simulink model "Md61Md62CalibSet"  (R2018b)
settings: Solver=FixedStepDiscrete  StartTime=0.0  StopTime=10.0  FixedStep=0.01  RelTol=1e-3
undefined symbols (not defined in the file or in its folder): KeSMSuFirstRwStBackPosDelta_Val, KeSMSuFirstRwStCushFoldPosDelta_Val, KeSMSuFirstRwStFwdBkwdPosDelta_Val, KeSMSuThrdRwCushFoldPosDelta_Val, KeSMSwAcsMd30PassStBkReclnUpwdDnwdPos1_Val, KeSMSwAcsMd30PassStBkReclnUpwdDnwdPos1Max_Val, KeSMSwAcsMd30PassStBkReclnUpwdDnwdPos1Min_Val, KeSMSwAcsMd30PassStFldUpwdDnwdPos1_Val, KeSMSwAcsMd30PassStFrwdBkwdPos1_Val, KeSMSwAcsMd30PassStFrwdBkwdPos1Max_Val, KeSMSwAcsMd30PassStFrwdBkwdPos1Min_Val, KeSMSwSeatBkLimitPos_Val, KeSMSwSeatBkLimitPosDelt_Val
libraries: StIsPosChkLib x2
(part 2 of 5)

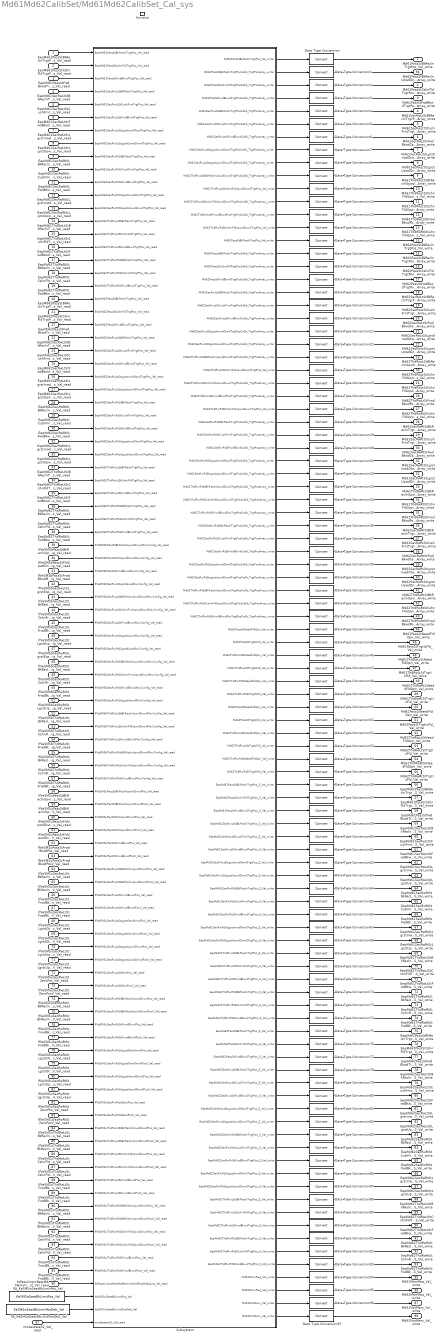
== system Md61Md62CalibSet/Md61Md62CalibSet_Cal_sys ==
  EepMd61PassStBkReclnTrgtPos_Val_read : Inport
  EepMd61PassStCshnFldTrgtPos_Val_read : Inport  Port=2
  EepMd61PassStFwdBkwdTrgtPos_Val_read : Inport  Port=3
  EepMd61SecRwLtStBkReclnTrgtPos_Val_read : Inport  Port=4
  EepMd61SecRwLtStCushFrntTrgtPos_Val_read : Inport  Port=5
  EepMd61SecRwLtStFwdBkwdTrgtPos_Val_read : Inport  Port=6
  EepMd61SecRwLtStLgrstInwdOtwdTrgtPos_Val_read : Inport  Port=7
  EepMd61SecRwLtStLgrstUpwdDnwdTrgtPos_Val_read : Inport  Port=8
  EepMd61SecRwRtStBkReclnTrgtPos_Val_read : Inport  Port=9
  EepMd61SecRwRtStCushFrntTrgtPos_Val_read : Inport  Port=10
  EepMd61SecRwRtStFwdBkwdTrgtPos_Val_read : Inport  Port=11
  EepMd61SecRwRtStLgrstInwdOtwdTrgtPos_Val_read : Inport  Port=12
  EepMd61SecRwRtStLgrstUpwdDnwdTrgtPos_Val_read : Inport  Port=13
  EepMd61ThdRwLtStBkReclnTrgtPos_Val_read : Inport  Port=14
  EepMd61ThdRwLtStCshnFldTrgtPos_Val_read : Inport  Port=15
  EepMd61ThdRwLtStFwdBkwdTrgtPos_Val_read : Inport  Port=16
  EepMd61ThdRwRtStBkReclnTrgtPos_Val_read : Inport  Port=17
  EepMd61ThdRwRtStCshnFldTrgtPos_Val_read : Inport  Port=18
  EepMd61ThdRwRtStFwdBkwdTrgtPos_Val_read : Inport  Port=19
  EepMd62PassStBkReclnTrgtPos_Val_read : Inport  Port=20
  EepMd62PassStCshnFldTrgtPos_Val_read : Inport  Port=21
  EepMd62PassStFwdBkwdTrgtPos_Val_read : Inport  Port=22
  EepMd62SecRwLtStBkReclnTrgtPos_Val_read : Inport  Port=23
  EepMd62SecRwLtStCushFrntTrgtPos_Val_read : Inport  Port=24
  EepMd62SecRwLtStFwdBkwdTrgtPos_Val_read : Inport  Port=25
  EepMd62SecRwLtStLgrstInwdOtwdTrgtPos_Val_read : Inport  Port=26
  EepMd62SecRwLtStLgrstUpwdDnwdTrgtPos_Val_read : Inport  Port=27
  EepMd62SecRwRtStBkReclnTrgtPos_Val_read : Inport  Port=28
  EepMd62SecRwRtStCushFrntTrgtPos_Val_read : Inport  Port=29
  EepMd62SecRwRtStFwdBkwdTrgtPos_Val_read : Inport  Port=30
  EepMd62SecRwRtStLgrstInwdOtwdTrgtPos_Val_read : Inport  Port=31
  EepMd62SecRwRtStLgrstUpwdDnwdTrgtPos_Val_read : Inport  Port=32
  EepMd62ThdRwLtStBkReclnTrgtPos_Val_read : Inport  Port=33
  EepMd62ThdRwLtStCshnFldTrgtPos_Val_read : Inport  Port=34
  EepMd62ThdRwLtStFwdBkwdTrgtPos_Val_read : Inport  Port=35
  EepMd62ThdRwRtStBkReclnTrgtPos_Val_read : Inport  Port=36
  EepMd62ThdRwRtStCshnFldTrgtPos_Val_read : Inport  Port=37
  EepMd62ThdRwRtStFwdBkwdTrgtPos_Val_read : Inport  Port=38
  IfVeSMSbPassStBkReclnUpwdDnwdMovConfig_Val_read : Inport  Port=39
  IfVeSMSbPassStFldUpwdDnwdMovConfig_Val_read : Inport  Port=40
  IfVeSMSbPassStFrwdBkwdMovConfig_Val_read : Inport  Port=41
  IfVeSMSbSecRwLtSLgrstExpdMovConfig_Val_read : Inport  Port=42
  IfVeSMSbSecRwLtStBkReclnUpwdDnwdMovConfig_Val_read : Inport  Port=43
  IfVeSMSbSecRwLtStCshnFrntUpwdDnwdMovConfig_Val_read : Inport  Port=44
  IfVeSMSbSecRwLtStFrwdBkwdMovConfig_Val_read : Inport  Port=45
  IfVeSMSbSecRwLtStLgrstUpwdMovConfig_Val_read : Inport  Port=46
  IfVeSMSbSecRwRtSLgrstExpdMovConfig_Val_read : Inport  Port=47
  IfVeSMSbSecRwRtStBkReclnUpwdDnwdMovConfig_Val_read : Inport  Port=48
  IfVeSMSbSecRwRtStCshnFrntUpwdDnwdMovConfig_Val_read : Inport  Port=49
  IfVeSMSbSecRwRtStFrwdBkwdMovConfig_Val_read : Inport  Port=50
  IfVeSMSbSecRwRtStLgrstUpwdMovConfig_Val_read : Inport  Port=51
  IfVeSMSbThdRwLtStBkReclnUpwdDnwdMovConfig_Val_read : Inport  Port=52
  IfVeSMSbThdRwLtStCshnFldUpwdDnwdMovConfig_Val_read : Inport  Port=53
  IfVeSMSbThdRwLtStFrwdBkwdMovConfig_Val_read : Inport  Port=54
  IfVeSMSbThdRwRtStBkReclnUpwdDnwdMovConfig_Val_read : Inport  Port=55
  IfVeSMSbThdRwRtStCshnFldUpwdDnwdMovConfig_Val_read : Inport  Port=56
  IfVeSMSbThdRwRtStFrwdBkwdMovConfig_Val_read : Inport  Port=57
  IfVeSMSuPassStBkReclnUpwdDnwdPos_Val_read : Inport  Port=58
  IfVeSMSuPassStBkReclnUpwdDnwdPosV_Val_read : Inport  Port=59
  IfVeSMSuPassStFldUpwdDnwdPos_Val_read : Inport  Port=60
  IfVeSMSuPassStFldUpwdDnwdPosV_Val_read : Inport  Port=61
  IfVeSMSuPassStFrwdBkwdPos_Val_read : Inport  Port=62
  IfVeSMSuPassStFrwdBkwdPosV_Val_read : Inport  Port=63
  IfVeSMSuSecRwLtStBkReclnUpwdDnwdPos_Val_read : Inport  Port=64
  IfVeSMSuSecRwLtStBkReclnUpwdDnwdPosV_Val_read : Inport  Port=65
  IfVeSMSuSecRwLtStFrwdBkwdPos_Val_read : Inport  Port=66
  IfVeSMSuSecRwLtStFrwdBkwdPosV_Val_read : Inport  Port=67
  IfVeSMSuSecRwLtStLgrstOtwdInwdPos_Val_read : Inport  Port=68
  IfVeSMSuSecRwLtStLgrstOtwdInwdPosV_Val_read : Inport  Port=69
  IfVeSMSuSecRwLtStLgrstUpwdDnwdPos_Val_read : Inport  Port=70
  IfVeSMSuSecRwLtStLgrstUpwdDnwdPosV_Val_read : Inport  Port=71
  IfVeSMSuSecRwLtStZeroPos_Val_read : Inport  Port=72
  IfVeSMSuSecRwLtStZeroPosV_Val_read : Inport  Port=73
  IfVeSMSuSecRwRtStBkReclnUpwdDnwdPos_Val_read : Inport  Port=74
  IfVeSMSuSecRwRtStBkReclnUpwdDnwdPosV_Val_read : Inport  Port=75
  IfVeSMSuSecRwRtStFrwdBkwdPos_Val_read : Inport  Port=76
  IfVeSMSuSecRwRtStFrwdBkwdPosV_Val_read : Inport  Port=77
  IfVeSMSuSecRwRtStLgrstOtwdInwdPos_Val_read : Inport  Port=78
  IfVeSMSuSecRwRtStLgrstOtwdInwdPosV_Val_read : Inport  Port=79
  IfVeSMSuSecRwRtStLgrstUpwdDnwdPos_Val_read : Inport  Port=80
  IfVeSMSuSecRwRtStLgrstUpwdDnwdPosV_Val_read : Inport  Port=81
  IfVeSMSuSecRwRtStZeroPos_Val_read : Inport  Port=82
  IfVeSMSuSecRwRtStZeroPosV_Val_read : Inport  Port=83
  IfVeSMSuThdRwLtStBkReclnUpwdDnwdPos_Val_read : Inport  Port=84
  IfVeSMSuThdRwLtStBkReclnUpwdDnwdPosV_Val_read : Inport  Port=85
  IfVeSMSuThdRwLtStCshnFldUpwdDnwdPos_Val_read : Inport  Port=86
  IfVeSMSuThdRwLtStCshnFldUpwdDnwdPosV_Val_read : Inport  Port=87
  IfVeSMSuThdRwLtStFrwdBkwdPos_Val_read : Inport  Port=88
  IfVeSMSuThdRwLtStFrwdBkwdPosV_Val_read : Inport  Port=89
  IfVeSMSuThdRwRtStBkReclnUpwdDnwdPos_Val_read : Inport  Port=90
  IfVeSMSuThdRwRtStBkReclnUpwdDnwdPosV_Val_read : Inport  Port=91
  IfVeSMSuThdRwRtStCshnFldUpwdDnwdPos_Val_read : Inport  Port=92
  IfVeSMSuThdRwRtStCshnFldUpwdDnwdPosV_Val_read : Inport  Port=93
  IfVeSMSuThdRwRtStFrwdBkwdPos_Val_read : Inport  Port=94
  IfVeSMSuThdRwRtStFrwdBkwdPosV_Val_read : Inport  Port=95
  StPassCmprtRestMdMemVirtCtrlReqMdadjust_Val_read : Inport  Port=96
  modestate32_Val_read : Inport  Port=97
  function : TriggerPort  TriggerType=function-call  IsSimulinkFunction=on  FunctionName=Md61Md62CalibSet_Cal  VariantControl=(inherit)
  Data Type Conversion{,1..97} (98 alike) : DataTypeConversion
  PA_KeSMSwSeatBkLimitPosDelt_Val : Constant  Value=KeSMSwSeatBkLimitPosDelt_Val
  PA_KeSMSwSeatBkLimitPos_Val : Constant  Value=KeSMSwSeatBkLimitPos_Val
  Subsystem : Subsystem
  Md61PassStBkReclnTrgtPos_Val_write : Outport
      settings: EnsureOutportIsVirtual=on
  Md61PassStCshnFldTrgtPosCalib_TrgtPosArray_write : Outport  Port=2
      settings: EnsureOutportIsVirtual=on
  Md61PassStFwdBkwdTrgtPosCalib_TrgtPosArray_write : Outport  Port=3
      settings: EnsureOutportIsVirtual=on
  Md61SecRwLtStBkReclnTrgtPosCalib_TrgtPosArray_write : Outport  Port=4
      settings: EnsureOutportIsVirtual=on
  Md61SecRwLtStCushFrntTrgtPosCalib_TrgtPosArray_write : Outport  Port=5
      settings: EnsureOutportIsVirtual=on
  Md61SecRwLtStFwdBkwdCalib_TrgtPosArray_write : Outport  Port=6
      settings: EnsureOutportIsVirtual=on
  Md61SecRwLtStLgrstInwdOtwdTrgtPosCalib_TrgtPosArray_write : Outport  Port=7
      settings: EnsureOutportIsVirtual=on
  Md61SecRwLtStLgrstUpwdDnwdTrgtPosCalib_TrgtPosArray_write : Outport  Port=8
      settings: EnsureOutportIsVirtual=on
  Md61ThdRwLtStBkReclnUpwdDnwdTrgtPosCalib_TrgtPosArray_write : Outport  Port=9
      settings: EnsureOutportIsVirtual=on
  Md61ThdRwLtStCshnFldUpwdDnwdTrgtPos_Val_write : Outport  Port=10
      settings: EnsureOutportIsVirtual=on
  Md61ThdRwLtStCshnFldUpwdDnwdTrgtPosCalib_TrgtPosArray_write : Outport  Port=11
      settings: EnsureOutportIsVirtual=on
  Md61ThdRwLtStFrwdBkwdPosTrgtPosCalib_TrgtPosArray_write : Outport  Port=12
      settings: EnsureOutportIsVirtual=on
  Md61ThdRwRtStCshnFldUpwdDnwdTrgtPos_Val_write : Outport  Port=13
      settings: EnsureOutportIsVirtual=on
  Md62PassStBkReclnTrgtPos_Val_write : Outport  Port=14
      settings: EnsureOutportIsVirtual=on
  Md62PassStBkReclnTrgtPosCalib_TrgtPosArray_write : Outport  Port=15
      settings: EnsureOutportIsVirtual=on
  Md62PassStCshnFldTrgtPosCalib_TrgtPosArray_write : Outport  Port=16
      settings: EnsureOutportIsVirtual=on
  Md62PassStFwdBkwdTrgtPosCalib_TrgtPosArray_write : Outport  Port=17
      settings: EnsureOutportIsVirtual=on
  Md62SecRwLtStBkReclnTrgtPosCalib_TrgtPosArray_write : Outport  Port=18
      settings: EnsureOutportIsVirtual=on
  Md62SecRwLtStCushFrntTrgtPosCalib_TrgtPosArray_write : Outport  Port=19
      settings: EnsureOutportIsVirtual=on
  Md62SecRwLtStFwdBkwdCalib_TrgtPosArray_write : Outport  Port=20
      settings: EnsureOutportIsVirtual=on
  Md62SecRwLtStLgrstInwdOtwdTrgtPosCalib_TrgtPosArray_write : Outport  Port=21
      settings: EnsureOutportIsVirtual=on
  Md62SecRwLtStLgrstUpwdDnwdTrgtPosCalib_TrgtPosArray_write : Outport  Port=22
      settings: EnsureOutportIsVirtual=on
  Md62ThdRwLtStBkReclnUpwdDnwdTrgtPosCalib_TrgtPosArray_write : Outport  Port=23
      settings: EnsureOutportIsVirtual=on
  Md62ThdRwLtStCshnFldUpwdDnwdTrgtPos_Val_write : Outport  Port=24
      settings: EnsureOutportIsVirtual=on
  Md62ThdRwLtStCshnFldUpwdDnwdTrgtPosCalib_TrgtPosArray_write : Outport  Port=25
      settings: EnsureOutportIsVirtual=on
  Md62ThdRwLtStFrwdBkwdPosTrgtPosCalib_TrgtPosArray_write : Outport  Port=26
      settings: EnsureOutportIsVirtual=on
  Md62ThdRwRtStCshnFldUpwdDnwdTrgtPos_Val_write : Outport  Port=27
      settings: EnsureOutportIsVirtual=on
  Md61SecRwRtStBkReclnTrgtPosCalib_TrgtPosArray_write : Outport  Port=28
      settings: EnsureOutportIsVirtual=on
  Md61SecRwRtStCushFrntTrgtPosCalib_TrgtPosArray_write : Outport  Port=29
      settings: EnsureOutportIsVirtual=on
  Md61SecRwRtStFwdBkwdCalib_TrgtPosArray_write : Outport  Port=30
      settings: EnsureOutportIsVirtual=on
  Md61SecRwRtStLgrstInwdOtwdTrgtPosCalib_TrgtPosArray_write : Outport  Port=31
      settings: EnsureOutportIsVirtual=on
  Md61SecRwRtStLgrstUpwdDnwdTrgtPosCalib_TrgtPosArray_write : Outport  Port=32
      settings: EnsureOutportIsVirtual=on
  Md61ThdRwRtStBkReclnUpwdDnwdTrgtPosCalib_TrgtPosArray_write : Outport  Port=33
      settings: EnsureOutportIsVirtual=on
  Md61ThdRwRtStCshnFldUpwdDnwdTrgtPosCalib_TrgtPosArray_write : Outport  Port=34
      settings: EnsureOutportIsVirtual=on
  Md61ThdRwRtStFrwdBkwdPosTrgtPosCalib_TrgtPosArray_write : Outport  Port=35
      settings: EnsureOutportIsVirtual=on
  Md62SecRwRtStBkReclnTrgtPosCalib_TrgtPosArray_write : Outport  Port=36
      settings: EnsureOutportIsVirtual=on
  Md62SecRwRtStCushFrntTrgtPosCalib_TrgtPosArray_write : Outport  Port=37
      settings: EnsureOutportIsVirtual=on
  Md62SecRwRtStFwdBkwdCalib_TrgtPosArray_write : Outport  Port=38
      settings: EnsureOutportIsVirtual=on
  Md62SecRwRtStLgrstInwdOtwdTrgtPosCalib_TrgtPosArray_write : Outport  Port=39
      settings: EnsureOutportIsVirtual=on
  Md62SecRwRtStLgrstUpwdDnwdTrgtPosCalib_TrgtPosArray_write : Outport  Port=40
      settings: EnsureOutportIsVirtual=on
  Md62ThdRwRtStBkReclnUpwdDnwdTrgtPosCalib_TrgtPosArray_write : Outport  Port=41
      settings: EnsureOutportIsVirtual=on
  Md62ThdRwRtStCshnFldUpwdDnwdTrgtPosCalib_TrgtPosArray_write : Outport  Port=42
      settings: EnsureOutportIsVirtual=on
  Md62ThdRwRtStFrwdBkwdPosTrgtPosCalib_TrgtPosArray_write : Outport  Port=43
      settings: EnsureOutportIsVirtual=on
  Md61PassStNeedFldOpn_Val_write : Outport  Port=44
      settings: EnsureOutportIsVirtual=on
  Md61PassStTrgtIsFld_Val_write : Outport  Port=45
      settings: EnsureOutportIsVirtual=on
  Md61ThdRwLtStNeedFldOpn_Val_write : Outport  Port=46
      settings: EnsureOutportIsVirtual=on
  Md61ThdRwLtStTrgtIsFld_Val_write : Outport  Port=47
      settings: EnsureOutportIsVirtual=on
  Md61ThdRwRtStNeedFldOpn_Val_write : Outport  Port=48
      settings: EnsureOutportIsVirtual=on
  Md61ThdRwRtStTrgtIsFld_Val_write : Outport  Port=49
      settings: EnsureOutportIsVirtual=on
  Md62PassStNeedFldOpn_Val_write : Outport  Port=50
      settings: EnsureOutportIsVirtual=on
  Md62PassStTrgtIsFld_Val_write : Outport  Port=51
      settings: EnsureOutportIsVirtual=on
  Md62ThdRwLtStNeedFldOpn_Val_write : Outport  Port=52
      settings: EnsureOutportIsVirtual=on
  Md62ThdRwLtStTrgtIsFld_Val_write : Outport  Port=53
      settings: EnsureOutportIsVirtual=on
  Md62ThdRwRtStNeedFldOpn_Val_write : Outport  Port=54
      settings: EnsureOutportIsVirtual=on
  Md62ThdRwRtStTrgtIsFld_Val_write : Outport  Port=55
      settings: EnsureOutportIsVirtual=on
  EepMd61PassStBkReclnTrgtPos_S_Val_write : Outport  Port=56
      settings: EnsureOutportIsVirtual=on
  EepMd61PassStCshnFldTrgtPos_S_Val_write : Outport  Port=57
      settings: EnsureOutportIsVirtual=on
  EepMd61PassStFwdBkwdTrgtPos_S_Val_write : Outport  Port=58
      settings: EnsureOutportIsVirtual=on
  EepMd61SecRwLtStBkReclnTrgtPos_S_Val_write : Outport  Port=59
      settings: EnsureOutportIsVirtual=on
  EepMd61SecRwLtStCushFrntTrgtPos_S_Val_write : Outport  Port=60
      settings: EnsureOutportIsVirtual=on
  EepMd61SecRwLtStFwdBkwdTrgtPos_S_Val_write : Outport  Port=61
      settings: EnsureOutportIsVirtual=on
  EepMd61SecRwLtStLgrstInwdOtwdTrgtPos_S_Val_write : Outport  Port=62
      settings: EnsureOutportIsVirtual=on
  EepMd61SecRwLtStLgrstUpwdDnwdTrgtPos_S_Val_write : Outport  Port=63
      settings: EnsureOutportIsVirtual=on
  EepMd61SecRwRtStBkReclnTrgtPos_S_Val_write : Outport  Port=64
      settings: EnsureOutportIsVirtual=on
  EepMd61SecRwRtStCushFrntTrgtPos_S_Val_write : Outport  Port=65
      settings: EnsureOutportIsVirtual=on
  EepMd61SecRwRtStFwdBkwdTrgtPos_S_Val_write : Outport  Port=66
      settings: EnsureOutportIsVirtual=on
  EepMd61SecRwRtStLgrstInwdOtwdTrgtPos_S_Val_write : Outport  Port=67
      settings: EnsureOutportIsVirtual=on
  EepMd61SecRwRtStLgrstUpwdDnwdTrgtPos_S_Val_write : Outport  Port=68
      settings: EnsureOutportIsVirtual=on
  EepMd61ThdRwLtStBkReclnTrgtPos_S_Val_write : Outport  Port=69
      settings: EnsureOutportIsVirtual=on
  EepMd61ThdRwLtStCshnFldTrgtPos_S_Val_write : Outport  Port=70
      settings: EnsureOutportIsVirtual=on
  EepMd61ThdRwLtStFwdBkwdTrgtPos_S_Val_write : Outport  Port=71
      settings: EnsureOutportIsVirtual=on
  EepMd61ThdRwRtStBkReclnTrgtPos_S_Val_write : Outport  Port=72
      settings: EnsureOutportIsVirtual=on
  EepMd61ThdRwRtStCshnFldTrgtPos_S_Val_write : Outport  Port=73
      settings: EnsureOutportIsVirtual=on
  EepMd61ThdRwRtStFwdBkwdTrgtPos_S_Val_write : Outport  Port=74
      settings: EnsureOutportIsVirtual=on
  EepMd62PassStBkReclnTrgtPos_S_Val_write : Outport  Port=75
      settings: EnsureOutportIsVirtual=on
  EepMd62PassStCshnFldTrgtPos_S_Val_write : Outport  Port=76
      settings: EnsureOutportIsVirtual=on
  EepMd62PassStFwdBkwdTrgtPos_S_Val_write : Outport  Port=77
      settings: EnsureOutportIsVirtual=on
  EepMd62SecRwLtStBkReclnTrgtPos_S_Val_write : Outport  Port=78
      settings: EnsureOutportIsVirtual=on
  EepMd62SecRwLtStCushFrntTrgtPos_S_Val_write : Outport  Port=79
      settings: EnsureOutportIsVirtual=on
  EepMd62SecRwLtStFwdBkwdTrgtPos_S_Val_write : Outport  Port=80
      settings: EnsureOutportIsVirtual=on
  EepMd62SecRwLtStLgrstInwdOtwdTrgtPos_S_Val_write : Outport  Port=81
      settings: EnsureOutportIsVirtual=on
  EepMd62SecRwLtStLgrstUpwdDnwdTrgtPos_S_Val_write : Outport  Port=82
      settings: EnsureOutportIsVirtual=on
  EepMd62SecRwRtStBkReclnTrgtPos_S_Val_write : Outport  Port=83
      settings: EnsureOutportIsVirtual=on
  EepMd62SecRwRtStCushFrntTrgtPos_S_Val_write : Outport  Port=84
      settings: EnsureOutportIsVirtual=on
  EepMd62SecRwRtStFwdBkwdTrgtPos_S_Val_write : Outport  Port=85
      settings: EnsureOutportIsVirtual=on
  EepMd62SecRwRtStLgrstInwdOtwdTrgtPos_S_Val_write : Outport  Port=86
      settings: EnsureOutportIsVirtual=on
  EepMd62SecRwRtStLgrstUpwdDnwdTrgtPos_S_Val_write : Outport  Port=87
      settings: EnsureOutportIsVirtual=on
  EepMd62ThdRwLtStBkReclnTrgtPos_S_Val_write : Outport  Port=88
      settings: EnsureOutportIsVirtual=on
  EepMd62ThdRwLtStCshnFldTrgtPos_S_Val_write : Outport  Port=89
      settings: EnsureOutportIsVirtual=on
  EepMd62ThdRwLtStFwdBkwdTrgtPos_S_Val_write : Outport  Port=90
      settings: EnsureOutportIsVirtual=on
  EepMd62ThdRwRtStBkReclnTrgtPos_S_Val_write : Outport  Port=91
      settings: EnsureOutportIsVirtual=on
  EepMd62ThdRwRtStCshnFldTrgtPos_S_Val_write : Outport  Port=92
      settings: EnsureOutportIsVirtual=on
  EepMd62ThdRwRtStFwdBkwdTrgtPos_S_Val_write : Outport  Port=93
      settings: EnsureOutportIsVirtual=on
  Md61PassStBkReclnUpwdDnwdTrgtPosCalib_TrgtPosArray_write : Outport  Port=94
      settings: EnsureOutportIsVirtual=on
  Md61MemReq_Val_write : Outport  Port=95
      settings: EnsureOutportIsVirtual=on
  Md62MemReq_Val_write : Outport  Port=96
      settings: EnsureOutportIsVirtual=on
  Md61NotMem_Val_write : Outport  Port=97
      settings: EnsureOutportIsVirtual=on
  Md62NotMem_Val_write : Outport  Port=98
      settings: EnsureOutportIsVirtual=on
  wires:
  EepMd61PassStBkReclnTrgtPos_Val_read/1 -> Subsystem/1(EepMd61PassStBkReclnTrgtPos_Val_read)
  EepMd61PassStCshnFldTrgtPos_Val_read/1 -> Subsystem/2(EepMd61PassStCshnFldTrgtPos_Val_read)
  EepMd61PassStFwdBkwdTrgtPos_Val_read/1 -> Subsystem/3(EepMd61PassStFwdBkwdTrgtPos_Val_read)
  EepMd61SecRwLtStBkReclnTrgtPos_Val_read/1 -> Subsystem/4(EepMd61SecRwLtStBkReclnTrgtPos_Val_read)
  EepMd61SecRwLtStCushFrntTrgtPos_Val_read/1 -> Subsystem/5(EepMd61SecRwLtStCushFrntTrgtPos_Val_read)
  EepMd61SecRwLtStFwdBkwdTrgtPos_Val_read/1 -> Subsystem/6(EepMd61SecRwLtStFwdBkwdTrgtPos_Val_read)
  EepMd61SecRwLtStLgrstInwdOtwdTrgtPos_Val_read/1 -> Subsystem/7(EepMd61SecRwLtStLgrstInwdOtwdTrgtPos_Val_read)
  EepMd61SecRwLtStLgrstUpwdDnwdTrgtPos_Val_read/1 -> Subsystem/8(EepMd61SecRwLtStLgrstUpwdDnwdTrgtPos_Val_read)
  EepMd61SecRwRtStBkReclnTrgtPos_Val_read/1 -> Subsystem/9(EepMd61SecRwRtStBkReclnTrgtPos_Val_read)
  EepMd61SecRwRtStCushFrntTrgtPos_Val_read/1 -> Subsystem/10(EepMd61SecRwRtStCushFrntTrgtPos_Val_read)
  EepMd61SecRwRtStFwdBkwdTrgtPos_Val_read/1 -> Subsystem/11(EepMd61SecRwRtStFwdBkwdTrgtPos_Val_read)
  EepMd61SecRwRtStLgrstInwdOtwdTrgtPos_Val_read/1 -> Subsystem/12(EepMd61SecRwRtStLgrstInwdOtwdTrgtPos_Val_read)
  EepMd61SecRwRtStLgrstUpwdDnwdTrgtPos_Val_read/1 -> Subsystem/13(EepMd61SecRwRtStLgrstUpwdDnwdTrgtPos_Val_read)
  EepMd61ThdRwLtStBkReclnTrgtPos_Val_read/1 -> Subsystem/14(EepMd61ThdRwLtStBkReclnTrgtPos_Val_read)
  EepMd61ThdRwLtStCshnFldTrgtPos_Val_read/1 -> Subsystem/15(EepMd61ThdRwLtStCshnFldTrgtPos_Val_read)
  EepMd61ThdRwLtStFwdBkwdTrgtPos_Val_read/1 -> Subsystem/16(EepMd61ThdRwLtStFwdBkwdTrgtPos_Val_read)
  EepMd61ThdRwRtStBkReclnTrgtPos_Val_read/1 -> Subsystem/17(EepMd61ThdRwRtStBkReclnTrgtPos_Val_read)
  EepMd61ThdRwRtStCshnFldTrgtPos_Val_read/1 -> Subsystem/18(EepMd61ThdRwRtStCshnFldTrgtPos_Val_read)
  EepMd61ThdRwRtStFwdBkwdTrgtPos_Val_read/1 -> Subsystem/19(EepMd61ThdRwRtStFwdBkwdTrgtPos_Val_read)
  EepMd62PassStBkReclnTrgtPos_Val_read/1 -> Subsystem/20(EepMd62PassStBkReclnTrgtPos_Val_read)
  EepMd62PassStCshnFldTrgtPos_Val_read/1 -> Subsystem/21(EepMd62PassStCshnFldTrgtPos_Val_read)
  EepMd62PassStFwdBkwdTrgtPos_Val_read/1 -> Subsystem/22(EepMd62PassStFwdBkwdTrgtPos_Val_read)
  EepMd62SecRwLtStBkReclnTrgtPos_Val_read/1 -> Subsystem/23(EepMd62SecRwLtStBkReclnTrgtPos_Val_read)
  EepMd62SecRwLtStCushFrntTrgtPos_Val_read/1 -> Subsystem/24(EepMd62SecRwLtStCushFrntTrgtPos_Val_read)
  EepMd62SecRwLtStFwdBkwdTrgtPos_Val_read/1 -> Subsystem/25(EepMd62SecRwLtStFwdBkwdTrgtPos_Val_read)
  EepMd62SecRwLtStLgrstInwdOtwdTrgtPos_Val_read/1 -> Subsystem/26(EepMd62SecRwLtStLgrstInwdOtwdTrgtPos_Val_read)
  EepMd62SecRwLtStLgrstUpwdDnwdTrgtPos_Val_read/1 -> Subsystem/27(EepMd62SecRwLtStLgrstUpwdDnwdTrgtPos_Val_read)
  EepMd62SecRwRtStBkReclnTrgtPos_Val_read/1 -> Subsystem/28(EepMd62SecRwRtStBkReclnTrgtPos_Val_read)
  EepMd62SecRwRtStCushFrntTrgtPos_Val_read/1 -> Subsystem/29(EepMd62SecRwRtStCushFrntTrgtPos_Val_read)
  EepMd62SecRwRtStFwdBkwdTrgtPos_Val_read/1 -> Subsystem/30(EepMd62SecRwRtStFwdBkwdTrgtPos_Val_read)
  EepMd62SecRwRtStLgrstInwdOtwdTrgtPos_Val_read/1 -> Subsystem/31(EepMd62SecRwRtStLgrstInwdOtwdTrgtPos_Val_read)
  EepMd62SecRwRtStLgrstUpwdDnwdTrgtPos_Val_read/1 -> Subsystem/32(EepMd62SecRwRtStLgrstUpwdDnwdTrgtPos_Val_read)
  EepMd62ThdRwLtStBkReclnTrgtPos_Val_read/1 -> Subsystem/33(EepMd62ThdRwLtStBkReclnTrgtPos_Val_read)
  EepMd62ThdRwLtStCshnFldTrgtPos_Val_read/1 -> Subsystem/34(EepMd62ThdRwLtStCshnFldTrgtPos_Val_read)
  EepMd62ThdRwLtStFwdBkwdTrgtPos_Val_read/1 -> Subsystem/35(EepMd62ThdRwLtStFwdBkwdTrgtPos_Val_read)
  EepMd62ThdRwRtStBkReclnTrgtPos_Val_read/1 -> Subsystem/36(EepMd62ThdRwRtStBkReclnTrgtPos_Val_read)
  EepMd62ThdRwRtStCshnFldTrgtPos_Val_read/1 -> Subsystem/37(EepMd62ThdRwRtStCshnFldTrgtPos_Val_read)
  EepMd62ThdRwRtStFwdBkwdTrgtPos_Val_read/1 -> Subsystem/38(EepMd62ThdRwRtStFwdBkwdTrgtPos_Val_read)
  IfVeSMSbPassStBkReclnUpwdDnwdMovConfig_Val_read/1 -> Subsystem/39(IfVeSMSbPassStBkReclnUpwdDnwdMovConfig_Val_read)
  IfVeSMSbPassStFldUpwdDnwdMovConfig_Val_read/1 -> Subsystem/40(IfVeSMSbPassStFldUpwdDnwdMovConfig_Val_read)
  IfVeSMSbPassStFrwdBkwdMovConfig_Val_read/1 -> Subsystem/41(IfVeSMSbPassStFrwdBkwdMovConfig_Val_read)
  IfVeSMSbSecRwLtSLgrstExpdMovConfig_Val_read/1 -> Subsystem/42(IfVeSMSbSecRwLtSLgrstExpdMovConfig_Val_read)
  IfVeSMSbSecRwLtStBkReclnUpwdDnwdMovConfig_Val_read/1 -> Subsystem/43(IfVeSMSbSecRwLtStBkReclnUpwdDnwdMovConfig_Val_read)
  IfVeSMSbSecRwLtStCshnFrntUpwdDnwdMovConfig_Val_read/1 -> Subsystem/44(IfVeSMSbSecRwLtStCshnFrntUpwdDnwdMovConfig_Val_read)
  IfVeSMSbSecRwLtStFrwdBkwdMovConfig_Val_read/1 -> Subsystem/45(IfVeSMSbSecRwLtStFrwdBkwdMovConfig_Val_read)
  IfVeSMSbSecRwLtStLgrstUpwdMovConfig_Val_read/1 -> Subsystem/46(IfVeSMSbSecRwLtStLgrstUpwdMovConfig_Val_read)
  IfVeSMSbSecRwRtSLgrstExpdMovConfig_Val_read/1 -> Subsystem/47(IfVeSMSbSecRwRtSLgrstExpdMovConfig_Val_read)
  IfVeSMSbSecRwRtStBkReclnUpwdDnwdMovConfig_Val_read/1 -> Subsystem/48(IfVeSMSbSecRwRtStBkReclnUpwdDnwdMovConfig_Val_read)
  IfVeSMSbSecRwRtStCshnFrntUpwdDnwdMovConfig_Val_read/1 -> Subsystem/49(IfVeSMSbSecRwRtStCshnFrntUpwdDnwdMovConfig_Val_read)
  IfVeSMSbSecRwRtStFrwdBkwdMovConfig_Val_read/1 -> Subsystem/50(IfVeSMSbSecRwRtStFrwdBkwdMovConfig_Val_read)
  IfVeSMSbSecRwRtStLgrstUpwdMovConfig_Val_read/1 -> Subsystem/51(IfVeSMSbSecRwRtStLgrstUpwdMovConfig_Val_read)
  IfVeSMSbThdRwLtStBkReclnUpwdDnwdMovConfig_Val_read/1 -> Subsystem/52(IfVeSMSbThdRwLtStBkReclnUpwdDnwdMovConfig_Val_read)
  IfVeSMSbThdRwLtStCshnFldUpwdDnwdMovConfig_Val_read/1 -> Subsystem/53(IfVeSMSbThdRwLtStCshnFldUpwdDnwdMovConfig_Val_read)
  IfVeSMSbThdRwLtStFrwdBkwdMovConfig_Val_read/1 -> Subsystem/54(IfVeSMSbThdRwLtStFrwdBkwdMovConfig_Val_read)
  IfVeSMSbThdRwRtStBkReclnUpwdDnwdMovConfig_Val_read/1 -> Subsystem/55(IfVeSMSbThdRwRtStBkReclnUpwdDnwdMovConfig_Val_read)
  IfVeSMSbThdRwRtStCshnFldUpwdDnwdMovConfig_Val_read/1 -> Subsystem/56(IfVeSMSbThdRwRtStCshnFldUpwdDnwdMovConfig_Val_read)
  IfVeSMSbThdRwRtStFrwdBkwdMovConfig_Val_read/1 -> Subsystem/57(IfVeSMSbThdRwRtStFrwdBkwdMovConfig_Val_read)
  IfVeSMSuPassStBkReclnUpwdDnwdPos_Val_read/1 -> Subsystem/58(IfVeSMSuPassStBkReclnUpwdDnwdPos_Val_read)
  IfVeSMSuPassStBkReclnUpwdDnwdPosV_Val_read/1 -> Subsystem/59(IfVeSMSuPassStBkReclnUpwdDnwdPosV_Val_read)
  IfVeSMSuPassStFldUpwdDnwdPos_Val_read/1 -> Subsystem/60(IfVeSMSuPassStFldUpwdDnwdPos_Val_read)
  IfVeSMSuPassStFldUpwdDnwdPosV_Val_read/1 -> Subsystem/61(IfVeSMSuPassStFldUpwdDnwdPosV_Val_read)
  IfVeSMSuPassStFrwdBkwdPos_Val_read/1 -> Subsystem/62(IfVeSMSuPassStFrwdBkwdPos_Val_read)
  IfVeSMSuPassStFrwdBkwdPosV_Val_read/1 -> Subsystem/63(IfVeSMSuPassStFrwdBkwdPosV_Val_read)
  IfVeSMSuSecRwLtStBkReclnUpwdDnwdPos_Val_read/1 -> Subsystem/64(IfVeSMSuSecRwLtStBkReclnUpwdDnwdPos_Val_read)
  IfVeSMSuSecRwLtStBkReclnUpwdDnwdPosV_Val_read/1 -> Subsystem/65(IfVeSMSuSecRwLtStBkReclnUpwdDnwdPosV_Val_read)
  IfVeSMSuSecRwLtStFrwdBkwdPos_Val_read/1 -> Subsystem/66(IfVeSMSuSecRwLtStFrwdBkwdPos_Val_read)
  IfVeSMSuSecRwLtStFrwdBkwdPosV_Val_read/1 -> Subsystem/67(IfVeSMSuSecRwLtStFrwdBkwdPosV_Val_read)
  IfVeSMSuSecRwLtStLgrstOtwdInwdPos_Val_read/1 -> Subsystem/68(IfVeSMSuSecRwLtStLgrstOtwdInwdPos_Val_read)
  IfVeSMSuSecRwLtStLgrstOtwdInwdPosV_Val_read/1 -> Subsystem/69(IfVeSMSuSecRwLtStLgrstOtwdInwdPosV_Val_read)
  IfVeSMSuSecRwLtStLgrstUpwdDnwdPos_Val_read/1 -> Subsystem/70(IfVeSMSuSecRwLtStLgrstUpwdDnwdPos_Val_read)
  IfVeSMSuSecRwLtStLgrstUpwdDnwdPosV_Val_read/1 -> Subsystem/71(IfVeSMSuSecRwLtStLgrstUpwdDnwdPosV_Val_read)
  IfVeSMSuSecRwLtStZeroPos_Val_read/1 -> Subsystem/72(IfVeSMSuSecRwLtStZeroPos_Val_read)
  IfVeSMSuSecRwLtStZeroPosV_Val_read/1 -> Subsystem/73(IfVeSMSuSecRwLtStZeroPosV_Val_read)
  IfVeSMSuSecRwRtStBkReclnUpwdDnwdPos_Val_read/1 -> Subsystem/74(IfVeSMSuSecRwRtStBkReclnUpwdDnwdPos_Val_read)
  IfVeSMSuSecRwRtStBkReclnUpwdDnwdPosV_Val_read/1 -> Subsystem/75(IfVeSMSuSecRwRtStBkReclnUpwdDnwdPosV_Val_read)
  IfVeSMSuSecRwRtStFrwdBkwdPos_Val_read/1 -> Subsystem/76(IfVeSMSuSecRwRtStFrwdBkwdPos_Val_read)
  IfVeSMSuSecRwRtStFrwdBkwdPosV_Val_read/1 -> Subsystem/77(IfVeSMSuSecRwRtStFrwdBkwdPosV_Val_read)
  IfVeSMSuSecRwRtStLgrstOtwdInwdPos_Val_read/1 -> Subsystem/78(IfVeSMSuSecRwRtStLgrstOtwdInwdPos_Val_read)
  IfVeSMSuSecRwRtStLgrstOtwdInwdPosV_Val_read/1 -> Subsystem/79(IfVeSMSuSecRwRtStLgrstOtwdInwdPosV_Val_read)
  IfVeSMSuSecRwRtStLgrstUpwdDnwdPos_Val_read/1 -> Subsystem/80(IfVeSMSuSecRwRtStLgrstUpwdDnwdPos_Val_read)
  IfVeSMSuSecRwRtStLgrstUpwdDnwdPosV_Val_read/1 -> Subsystem/81(IfVeSMSuSecRwRtStLgrstUpwdDnwdPosV_Val_read)
  IfVeSMSuSecRwRtStZeroPos_Val_read/1 -> Subsystem/82(IfVeSMSuSecRwRtStZeroPos_Val_read)
  IfVeSMSuSecRwRtStZeroPosV_Val_read/1 -> Subsystem/83(IfVeSMSuSecRwRtStZeroPosV_Val_read)
  IfVeSMSuThdRwLtStBkReclnUpwdDnwdPos_Val_read/1 -> Subsystem/84(IfVeSMSuThdRwLtStBkReclnUpwdDnwdPos_Val_read)
  IfVeSMSuThdRwLtStBkReclnUpwdDnwdPosV_Val_read/1 -> Subsystem/85(IfVeSMSuThdRwLtStBkReclnUpwdDnwdPosV_Val_read)
  IfVeSMSuThdRwLtStCshnFldUpwdDnwdPos_Val_read/1 -> Subsystem/86(IfVeSMSuThdRwLtStCshnFldUpwdDnwdPos_Val_read)
  IfVeSMSuThdRwLtStCshnFldUpwdDnwdPosV_Val_read/1 -> Subsystem/87(IfVeSMSuThdRwLtStCshnFldUpwdDnwdPosV_Val_read)
  IfVeSMSuThdRwLtStFrwdBkwdPos_Val_read/1 -> Subsystem/88(IfVeSMSuThdRwLtStFrwdBkwdPos_Val_read)
  IfVeSMSuThdRwLtStFrwdBkwdPosV_Val_read/1 -> Subsystem/89(IfVeSMSuThdRwLtStFrwdBkwdPosV_Val_read)
  IfVeSMSuThdRwRtStBkReclnUpwdDnwdPos_Val_read/1 -> Subsystem/90(IfVeSMSuThdRwRtStBkReclnUpwdDnwdPos_Val_read)
  IfVeSMSuThdRwRtStBkReclnUpwdDnwdPosV_Val_read/1 -> Subsystem/91(IfVeSMSuThdRwRtStBkReclnUpwdDnwdPosV_Val_read)
  IfVeSMSuThdRwRtStCshnFldUpwdDnwdPos_Val_read/1 -> Subsystem/92(IfVeSMSuThdRwRtStCshnFldUpwdDnwdPos_Val_read)
  IfVeSMSuThdRwRtStCshnFldUpwdDnwdPosV_Val_read/1 -> Subsystem/93(IfVeSMSuThdRwRtStCshnFldUpwdDnwdPosV_Val_read)
  IfVeSMSuThdRwRtStFrwdBkwdPos_Val_read/1 -> Subsystem/94(IfVeSMSuThdRwRtStFrwdBkwdPos_Val_read)
  IfVeSMSuThdRwRtStFrwdBkwdPosV_Val_read/1 -> Subsystem/95(IfVeSMSuThdRwRtStFrwdBkwdPosV_Val_read)
  StPassCmprtRestMdMemVirtCtrlReqMdadjust_Val_read/1 -> Subsystem/96(StPassCmprtRestMdMemVirtCtrlReqMdadjust_Val_read)
  Subsystem/1(Md61PassStBkReclnTrgtPos_Val_write) -> Data Type Conversion/1
  Subsystem/2(Md61PassStBkReclnTrgtPosCalib_TrgtPosArray_write) -> Data Type Conversion1/1
  Subsystem/3(Md61PassStCshnFldTrgtPosCalib_TrgtPosArray_write) -> Data Type Conversion2/1
  Subsystem/4(Md61PassStFwdBkwdTrgtPosCalib_TrgtPosArray_write) -> Data Type Conversion3/1
  Subsystem/5(Md61SecRwLtStBkReclnTrgtPosCalib_TrgtPosArray_write) -> Data Type Conversion4/1
  Subsystem/6(Md61SecRwLtStCushFrntTrgtPosCalib_TrgtPosArray_write) -> Data Type Conversion5/1
  Subsystem/7(Md61SecRwLtStFwdBkwdCalib_TrgtPosArray_write) -> Data Type Conversion6/1
  Subsystem/8(Md61SecRwLtStLgrstInwdOtwdTrgtPosCalib_TrgtPosArray_write) -> Data Type Conversion7/1
  Subsystem/9(Md61SecRwLtStLgrstUpwdDnwdTrgtPosCalib_TrgtPosArray_write) -> Data Type Conversion8/1
  Subsystem/10(Md61ThdRwLtStBkReclnUpwdDnwdTrgtPosCalib_TrgtPosArray_write) -> Data Type Conversion9/1
  Subsystem/11(Md61ThdRwLtStCshnFldUpwdDnwdTrgtPos_Val_write) -> Data Type Conversion10/1
  Subsystem/12(Md61ThdRwLtStCshnFldUpwdDnwdTrgtPosCalib_TrgtPosArray_write) -> Data Type Conversion11/1
  Subsystem/13(Md61ThdRwLtStFrwdBkwdPosTrgtPosCalib_TrgtPosArray_write) -> Data Type Conversion12/1
  Subsystem/14(Md61ThdRwRtStCshnFldUpwdDnwdTrgtPos_Val_write) -> Data Type Conversion13/1
  Subsystem/15(Md62PassStBkReclnTrgtPos_Val_write) -> Data Type Conversion14/1
  Subsystem/16(Md62PassStBkReclnTrgtPosCalib_TrgtPosArray_write) -> Data Type Conversion15/1
  Subsystem/17(Md62PassStCshnFldTrgtPosCalib_TrgtPosArray_write) -> Data Type Conversion16/1
  Subsystem/18(Md62PassStFwdBkwdTrgtPosCalib_TrgtPosArray_write) -> Data Type Conversion17/1
  Subsystem/19(Md62SecRwLtStBkReclnTrgtPosCalib_TrgtPosArray_write) -> Data Type Conversion18/1
  Subsystem/20(Md62SecRwLtStCushFrntTrgtPosCalib_TrgtPosArray_write) -> Data Type Conversion19/1
  Subsystem/21(Md62SecRwLtStFwdBkwdCalib_TrgtPosArray_write) -> Data Type Conversion20/1
  Subsystem/22(Md62SecRwLtStLgrstInwdOtwdTrgtPosCalib_TrgtPosArray_write) -> Data Type Conversion21/1
  Subsystem/23(Md62SecRwLtStLgrstUpwdDnwdTrgtPosCalib_TrgtPosArray_write) -> Data Type Conversion22/1
  Subsystem/24(Md62ThdRwLtStBkReclnUpwdDnwdTrgtPosCalib_TrgtPosArray_write) -> Data Type Conversion23/1
  Subsystem/25(Md62ThdRwLtStCshnFldUpwdDnwdTrgtPos_Val_write) -> Data Type Conversion24/1
  Subsystem/26(Md62ThdRwLtStCshnFldUpwdDnwdTrgtPosCalib_TrgtPosArray_write) -> Data Type Conversion25/1
  Subsystem/27(Md62ThdRwLtStFrwdBkwdPosTrgtPosCalib_TrgtPosArray_write) -> Data Type Conversion26/1
  Subsystem/28(Md62ThdRwRtStCshnFldUpwdDnwdTrgtPos_Val_write) -> Data Type Conversion27/1
  Subsystem/38(Md62SecRwRtStCushFrntTrgtPosCalib_TrgtPosArray_write) -> Data Type Conversion37/1
  Subsystem/39(Md62SecRwRtStFwdBkwdCalib_TrgtPosArray_write) -> Data Type Conversion38/1
  Subsystem/37(Md62SecRwRtStBkReclnTrgtPosCalib_TrgtPosArray_write) -> Data Type Conversion36/1
  Subsystem/36(Md61ThdRwRtStFrwdBkwdPosTrgtPosCalib_TrgtPosArray_write) -> Data Type Conversion35/1
  Subsystem/40(Md62SecRwRtStLgrstInwdOtwdTrgtPosCalib_TrgtPosArray_write) -> Data Type Conversion39/1
  Subsystem/35(Md61ThdRwRtStCshnFldUpwdDnwdTrgtPosCalib_TrgtPosArray_write) -> Data Type Conversion34/1
  Subsystem/41(Md62SecRwRtStLgrstUpwdDnwdTrgtPosCalib_TrgtPosArray_write) -> Data Type Conversion40/1
  Subsystem/42(Md62ThdRwRtStBkReclnUpwdDnwdTrgtPosCalib_TrgtPosArray_write) -> Data Type Conversion41/1
  Subsystem/34(Md61ThdRwRtStBkReclnUpwdDnwdTrgtPosCalib_TrgtPosArray_write) -> Data Type Conversion33/1
  Subsystem/33(Md61SecRwRtStLgrstUpwdDnwdTrgtPosCalib_TrgtPosArray_write) -> Data Type Conversion32/1
  Subsystem/43(Md62ThdRwRtStCshnFldUpwdDnwdTrgtPosCalib_TrgtPosArray_write) -> Data Type Conversion42/1
  Subsystem/44(Md62ThdRwRtStFrwdBkwdPosTrgtPosCalib_TrgtPosArray_write) -> Data Type Conversion43/1
  Subsystem/32(Md61SecRwRtStLgrstInwdOtwdTrgtPosCalib_TrgtPosArray_write) -> Data Type Conversion31/1
  Subsystem/31(Md61SecRwRtStFwdBkwdCalib_TrgtPosArray_write) -> Data Type Conversion30/1
  Subsystem/30(Md61SecRwRtStCushFrntTrgtPosCalib_TrgtPosArray_write) -> Data Type Conversion29/1
  Subsystem/29(Md61SecRwRtStBkReclnTrgtPosCalib_TrgtPosArray_write) -> Data Type Conversion28/1
  PA_KeSMSwSeatBkLimitPos_Val/1 -> Subsystem/97(KeSMSwSeatBkLimitPos_Val)
  PA_KeSMSwSeatBkLimitPosDelt_Val/1 -> Subsystem/98(KeSMSwSeatBkLimitPosDelt_Val)
  modestate32_Val_read/1 -> Subsystem/99(modestate32_Val_read)
  Subsystem/56(Md62ThdRwRtStTrgtIsFld_Val_write) -> Data Type Conversion55/1
  Subsystem/55(Md62ThdRwRtStNeedFldOpn_Val_write) -> Data Type Conversion54/1
  Subsystem/54(Md62ThdRwLtStTrgtIsFld_Val_write) -> Data Type Conversion53/1
  Subsystem/53(Md62ThdRwLtStNeedFldOpn_Val_write) -> Data Type Conversion52/1
  Subsystem/52(Md62PassStTrgtIsFld_Val_write) -> Data Type Conversion51/1
  Subsystem/51(Md62PassStNeedFldOpn_Val_write) -> Data Type Conversion50/1
  Subsystem/50(Md61ThdRwRtStTrgtIsFld_Val_write) -> Data Type Conversion49/1
  Subsystem/49(Md61ThdRwRtStNeedFldOpn_Val_write) -> Data Type Conversion48/1
  Subsystem/48(Md61ThdRwLtStTrgtIsFld_Val_write) -> Data Type Conversion47/1
  Subsystem/47(Md61ThdRwLtStNeedFldOpn_Val_write) -> Data Type Conversion46/1
  Subsystem/46(Md61PassStTrgtIsFld_Val_write) -> Data Type Conversion45/1
  Subsystem/45(Md61PassStNeedFldOpn_Val_write) -> Data Type Conversion44/1
  Subsystem/94(EepMd62ThdRwRtStFwdBkwdTrgtPos_S_Val_write) -> Data Type Conversion93/1
  Subsystem/92(EepMd62ThdRwRtStBkReclnTrgtPos_S_Val_write) -> Data Type Conversion91/1
  Subsystem/93(EepMd62ThdRwRtStCshnFldTrgtPos_S_Val_write) -> Data Type Conversion92/1
  Subsystem/89(EepMd62ThdRwLtStBkReclnTrgtPos_S_Val_write) -> Data Type Conversion88/1
  Subsystem/90(EepMd62ThdRwLtStCshnFldTrgtPos_S_Val_write) -> Data Type Conversion89/1
  Subsystem/91(EepMd62ThdRwLtStFwdBkwdTrgtPos_S_Val_write) -> Data Type Conversion90/1
  Subsystem/87(EepMd62SecRwRtStLgrstInwdOtwdTrgtPos_S_Val_write) -> Data Type Conversion86/1
  Subsystem/88(EepMd62SecRwRtStLgrstUpwdDnwdTrgtPos_S_Val_write) -> Data Type Conversion87/1
  Subsystem/84(EepMd62SecRwRtStBkReclnTrgtPos_S_Val_write) -> Data Type Conversion83/1
  Subsystem/85(EepMd62SecRwRtStCushFrntTrgtPos_S_Val_write) -> Data Type Conversion84/1
  Subsystem/86(EepMd62SecRwRtStFwdBkwdTrgtPos_S_Val_write) -> Data Type Conversion85/1
  Subsystem/82(EepMd62SecRwLtStLgrstInwdOtwdTrgtPos_S_Val_write) -> Data Type Conversion81/1
  Subsystem/83(EepMd62SecRwLtStLgrstUpwdDnwdTrgtPos_S_Val_write) -> Data Type Conversion82/1
  Subsystem/79(EepMd62SecRwLtStBkReclnTrgtPos_S_Val_write) -> Data Type Conversion78/1
  Subsystem/80(EepMd62SecRwLtStCushFrntTrgtPos_S_Val_write) -> Data Type Conversion79/1
  Subsystem/81(EepMd62SecRwLtStFwdBkwdTrgtPos_S_Val_write) -> Data Type Conversion80/1
  Subsystem/77(EepMd62PassStCshnFldTrgtPos_S_Val_write) -> Data Type Conversion76/1
  Subsystem/78(EepMd62PassStFwdBkwdTrgtPos_S_Val_write) -> Data Type Conversion77/1
  Subsystem/74(EepMd61ThdRwRtStCshnFldTrgtPos_S_Val_write) -> Data Type Conversion73/1
  Subsystem/75(EepMd61ThdRwRtStFwdBkwdTrgtPos_S_Val_write) -> Data Type Conversion74/1
  Subsystem/76(EepMd62PassStBkReclnTrgtPos_S_Val_write) -> Data Type Conversion75/1
  Subsystem/72(EepMd61ThdRwLtStFwdBkwdTrgtPos_S_Val_write) -> Data Type Conversion71/1
  Subsystem/73(EepMd61ThdRwRtStBkReclnTrgtPos_S_Val_write) -> Data Type Conversion72/1
  Subsystem/69(EepMd61SecRwRtStLgrstUpwdDnwdTrgtPos_S_Val_write) -> Data Type Conversion68/1
  Subsystem/70(EepMd61ThdRwLtStBkReclnTrgtPos_S_Val_write) -> Data Type Conversion69/1
  Subsystem/71(EepMd61ThdRwLtStCshnFldTrgtPos_S_Val_write) -> Data Type Conversion70/1
  Subsystem/67(EepMd61SecRwRtStFwdBkwdTrgtPos_S_Val_write) -> Data Type Conversion66/1
  Subsystem/68(EepMd61SecRwRtStLgrstInwdOtwdTrgtPos_S_Val_write) -> Data Type Conversion67/1
  Subsystem/64(EepMd61SecRwLtStLgrstUpwdDnwdTrgtPos_S_Val_write) -> Data Type Conversion63/1
  Subsystem/65(EepMd61SecRwRtStBkReclnTrgtPos_S_Val_write) -> Data Type Conversion64/1
  Subsystem/66(EepMd61SecRwRtStCushFrntTrgtPos_S_Val_write) -> Data Type Conversion65/1
  Subsystem/62(EepMd61SecRwLtStFwdBkwdTrgtPos_S_Val_write) -> Data Type Conversion61/1
  Subsystem/63(EepMd61SecRwLtStLgrstInwdOtwdTrgtPos_S_Val_write) -> Data Type Conversion62/1
  Subsystem/59(EepMd61PassStFwdBkwdTrgtPos_S_Val_write) -> Data Type Conversion58/1
  Subsystem/60(EepMd61SecRwLtStBkReclnTrgtPos_S_Val_write) -> Data Type Conversion59/1
  Subsystem/61(EepMd61SecRwLtStCushFrntTrgtPos_S_Val_write) -> Data Type Conversion60/1
  Subsystem/57(EepMd61PassStBkReclnTrgtPos_S_Val_write) -> Data Type Conversion56/1
  Subsystem/58(EepMd61PassStCshnFldTrgtPos_S_Val_write) -> Data Type Conversion57/1
  Subsystem/95(Md61MemReq_Val_write) -> Data Type Conversion94/1
  Subsystem/96(Md62MemReq_Val_write) -> Data Type Conversion95/1
  Subsystem/97(Md61NotMem_Val_write) -> Data Type Conversion96/1
  Subsystem/98(Md62NotMem_Val_write) -> Data Type Conversion97/1
  Data Type Conversion/1 -> Md61PassStBkReclnTrgtPos_Val_write/1
  Data Type Conversion1/1 -> Md61PassStBkReclnUpwdDnwdTrgtPosCalib_TrgtPosArray_write/1
  Data Type Conversion2/1 -> Md61PassStCshnFldTrgtPosCalib_TrgtPosArray_write/1
  Data Type Conversion3/1 -> Md61PassStFwdBkwdTrgtPosCalib_TrgtPosArray_write/1
  Data Type Conversion4/1 -> Md61SecRwLtStBkReclnTrgtPosCalib_TrgtPosArray_write/1
  Data Type Conversion5/1 -> Md61SecRwLtStCushFrntTrgtPosCalib_TrgtPosArray_write/1
  Data Type Conversion6/1 -> Md61SecRwLtStFwdBkwdCalib_TrgtPosArray_write/1
  Data Type Conversion7/1 -> Md61SecRwLtStLgrstInwdOtwdTrgtPosCalib_TrgtPosArray_write/1
  Data Type Conversion8/1 -> Md61SecRwLtStLgrstUpwdDnwdTrgtPosCalib_TrgtPosArray_write/1
  Data Type Conversion9/1 -> Md61ThdRwLtStBkReclnUpwdDnwdTrgtPosCalib_TrgtPosArray_write/1
  Data Type Conversion10/1 -> Md61ThdRwLtStCshnFldUpwdDnwdTrgtPos_Val_write/1
  Data Type Conversion11/1 -> Md61ThdRwLtStCshnFldUpwdDnwdTrgtPosCalib_TrgtPosArray_write/1
  Data Type Conversion12/1 -> Md61ThdRwLtStFrwdBkwdPosTrgtPosCalib_TrgtPosArray_write/1
  Data Type Conversion13/1 -> Md61ThdRwRtStCshnFldUpwdDnwdTrgtPos_Val_write/1
  Data Type Conversion14/1 -> Md62PassStBkReclnTrgtPos_Val_write/1
  Data Type Conversion15/1 -> Md62PassStBkReclnTrgtPosCalib_TrgtPosArray_write/1
  Data Type Conversion16/1 -> Md62PassStCshnFldTrgtPosCalib_TrgtPosArray_write/1
  Data Type Conversion17/1 -> Md62PassStFwdBkwdTrgtPosCalib_TrgtPosArray_write/1
  Data Type Conversion18/1 -> Md62SecRwLtStBkReclnTrgtPosCalib_TrgtPosArray_write/1
  Data Type Conversion19/1 -> Md62SecRwLtStCushFrntTrgtPosCalib_TrgtPosArray_write/1
  Data Type Conversion20/1 -> Md62SecRwLtStFwdBkwdCalib_TrgtPosArray_write/1
  Data Type Conversion21/1 -> Md62SecRwLtStLgrstInwdOtwdTrgtPosCalib_TrgtPosArray_write/1
  Data Type Conversion22/1 -> Md62SecRwLtStLgrstUpwdDnwdTrgtPosCalib_TrgtPosArray_write/1
  Data Type Conversion23/1 -> Md62ThdRwLtStBkReclnUpwdDnwdTrgtPosCalib_TrgtPosArray_write/1
  Data Type Conversion24/1 -> Md62ThdRwLtStCshnFldUpwdDnwdTrgtPos_Val_write/1
  Data Type Conversion25/1 -> Md62ThdRwLtStCshnFldUpwdDnwdTrgtPosCalib_TrgtPosArray_write/1
  Data Type Conversion26/1 -> Md62ThdRwLtStFrwdBkwdPosTrgtPosCalib_TrgtPosArray_write/1
  Data Type Conversion27/1 -> Md62ThdRwRtStCshnFldUpwdDnwdTrgtPos_Val_write/1
  Data Type Conversion28/1 -> Md61SecRwRtStBkReclnTrgtPosCalib_TrgtPosArray_write/1
  Data Type Conversion29/1 -> Md61SecRwRtStCushFrntTrgtPosCalib_TrgtPosArray_write/1
  Data Type Conversion30/1 -> Md61SecRwRtStFwdBkwdCalib_TrgtPosArray_write/1
  Data Type Conversion31/1 -> Md61SecRwRtStLgrstInwdOtwdTrgtPosCalib_TrgtPosArray_write/1
  Data Type Conversion32/1 -> Md61SecRwRtStLgrstUpwdDnwdTrgtPosCalib_TrgtPosArray_write/1
  Data Type Conversion33/1 -> Md61ThdRwRtStBkReclnUpwdDnwdTrgtPosCalib_TrgtPosArray_write/1
  Data Type Conversion34/1 -> Md61ThdRwRtStCshnFldUpwdDnwdTrgtPosCalib_TrgtPosArray_write/1
  Data Type Conversion35/1 -> Md61ThdRwRtStFrwdBkwdPosTrgtPosCalib_TrgtPosArray_write/1
  Data Type Conversion36/1 -> Md62SecRwRtStBkReclnTrgtPosCalib_TrgtPosArray_write/1
  Data Type Conversion37/1 -> Md62SecRwRtStCushFrntTrgtPosCalib_TrgtPosArray_write/1
  Data Type Conversion38/1 -> Md62SecRwRtStFwdBkwdCalib_TrgtPosArray_write/1
  Data Type Conversion39/1 -> Md62SecRwRtStLgrstInwdOtwdTrgtPosCalib_TrgtPosArray_write/1
  Data Type Conversion40/1 -> Md62SecRwRtStLgrstUpwdDnwdTrgtPosCalib_TrgtPosArray_write/1
  Data Type Conversion41/1 -> Md62ThdRwRtStBkReclnUpwdDnwdTrgtPosCalib_TrgtPosArray_write/1
  Data Type Conversion42/1 -> Md62ThdRwRtStCshnFldUpwdDnwdTrgtPosCalib_TrgtPosArray_write/1
  Data Type Conversion43/1 -> Md62ThdRwRtStFrwdBkwdPosTrgtPosCalib_TrgtPosArray_write/1
  Data Type Conversion44/1 -> Md61PassStNeedFldOpn_Val_write/1
  Data Type Conversion45/1 -> Md61PassStTrgtIsFld_Val_write/1
  Data Type Conversion46/1 -> Md61ThdRwLtStNeedFldOpn_Val_write/1
  Data Type Conversion47/1 -> Md61ThdRwLtStTrgtIsFld_Val_write/1
  Data Type Conversion48/1 -> Md61ThdRwRtStNeedFldOpn_Val_write/1
  Data Type Conversion49/1 -> Md61ThdRwRtStTrgtIsFld_Val_write/1
  Data Type Conversion50/1 -> Md62PassStNeedFldOpn_Val_write/1
  Data Type Conversion51/1 -> Md62PassStTrgtIsFld_Val_write/1
  Data Type Conversion52/1 -> Md62ThdRwLtStNeedFldOpn_Val_write/1
  Data Type Conversion53/1 -> Md62ThdRwLtStTrgtIsFld_Val_write/1
  Data Type Conversion54/1 -> Md62ThdRwRtStNeedFldOpn_Val_write/1
  Data Type Conversion55/1 -> Md62ThdRwRtStTrgtIsFld_Val_write/1
  Data Type Conversion56/1 -> EepMd61PassStBkReclnTrgtPos_S_Val_write/1
  Data Type Conversion57/1 -> EepMd61PassStCshnFldTrgtPos_S_Val_write/1
  Data Type Conversion58/1 -> EepMd61PassStFwdBkwdTrgtPos_S_Val_write/1
  Data Type Conversion59/1 -> EepMd61SecRwLtStBkReclnTrgtPos_S_Val_write/1
  Data Type Conversion60/1 -> EepMd61SecRwLtStCushFrntTrgtPos_S_Val_write/1
  Data Type Conversion61/1 -> EepMd61SecRwLtStFwdBkwdTrgtPos_S_Val_write/1
  Data Type Conversion62/1 -> EepMd61SecRwLtStLgrstInwdOtwdTrgtPos_S_Val_write/1
  Data Type Conversion63/1 -> EepMd61SecRwLtStLgrstUpwdDnwdTrgtPos_S_Val_write/1
  Data Type Conversion64/1 -> EepMd61SecRwRtStBkReclnTrgtPos_S_Val_write/1
  Data Type Conversion65/1 -> EepMd61SecRwRtStCushFrntTrgtPos_S_Val_write/1
  Data Type Conversion66/1 -> EepMd61SecRwRtStFwdBkwdTrgtPos_S_Val_write/1
  Data Type Conversion67/1 -> EepMd61SecRwRtStLgrstInwdOtwdTrgtPos_S_Val_write/1
  Data Type Conversion68/1 -> EepMd61SecRwRtStLgrstUpwdDnwdTrgtPos_S_Val_write/1
  Data Type Conversion69/1 -> EepMd61ThdRwLtStBkReclnTrgtPos_S_Val_write/1
  Data Type Conversion70/1 -> EepMd61ThdRwLtStCshnFldTrgtPos_S_Val_write/1
  Data Type Conversion71/1 -> EepMd61ThdRwLtStFwdBkwdTrgtPos_S_Val_write/1
  Data Type Conversion72/1 -> EepMd61ThdRwRtStBkReclnTrgtPos_S_Val_write/1
  Data Type Conversion73/1 -> EepMd61ThdRwRtStCshnFldTrgtPos_S_Val_write/1
  Data Type Conversion74/1 -> EepMd61ThdRwRtStFwdBkwdTrgtPos_S_Val_write/1
  Data Type Conversion75/1 -> EepMd62PassStBkReclnTrgtPos_S_Val_write/1
  Data Type Conversion76/1 -> EepMd62PassStCshnFldTrgtPos_S_Val_write/1
  Data Type Conversion77/1 -> EepMd62PassStFwdBkwdTrgtPos_S_Val_write/1
  Data Type Conversion78/1 -> EepMd62SecRwLtStBkReclnTrgtPos_S_Val_write/1
  Data Type Conversion79/1 -> EepMd62SecRwLtStCushFrntTrgtPos_S_Val_write/1
  Data Type Conversion80/1 -> EepMd62SecRwLtStFwdBkwdTrgtPos_S_Val_write/1
  Data Type Conversion81/1 -> EepMd62SecRwLtStLgrstInwdOtwdTrgtPos_S_Val_write/1
  Data Type Conversion82/1 -> EepMd62SecRwLtStLgrstUpwdDnwdTrgtPos_S_Val_write/1
  Data Type Conversion83/1 -> EepMd62SecRwRtStBkReclnTrgtPos_S_Val_write/1
  Data Type Conversion84/1 -> EepMd62SecRwRtStCushFrntTrgtPos_S_Val_write/1
  Data Type Conversion85/1 -> EepMd62SecRwRtStFwdBkwdTrgtPos_S_Val_write/1
  Data Type Conversion86/1 -> EepMd62SecRwRtStLgrstInwdOtwdTrgtPos_S_Val_write/1
  Data Type Conversion87/1 -> EepMd62SecRwRtStLgrstUpwdDnwdTrgtPos_S_Val_write/1
  Data Type Conversion88/1 -> EepMd62ThdRwLtStBkReclnTrgtPos_S_Val_write/1
  Data Type Conversion89/1 -> EepMd62ThdRwLtStCshnFldTrgtPos_S_Val_write/1
  Data Type Conversion90/1 -> EepMd62ThdRwLtStFwdBkwdTrgtPos_S_Val_write/1
  Data Type Conversion91/1 -> EepMd62ThdRwRtStBkReclnTrgtPos_S_Val_write/1
  Data Type Conversion92/1 -> EepMd62ThdRwRtStCshnFldTrgtPos_S_Val_write/1
  Data Type Conversion93/1 -> EepMd62ThdRwRtStFwdBkwdTrgtPos_S_Val_write/1
  Data Type Conversion94/1 -> Md61MemReq_Val_write/1
  Data Type Conversion95/1 -> Md62MemReq_Val_write/1
  Data Type Conversion96/1 -> Md61NotMem_Val_write/1
  Data Type Conversion97/1 -> Md62NotMem_Val_write/1

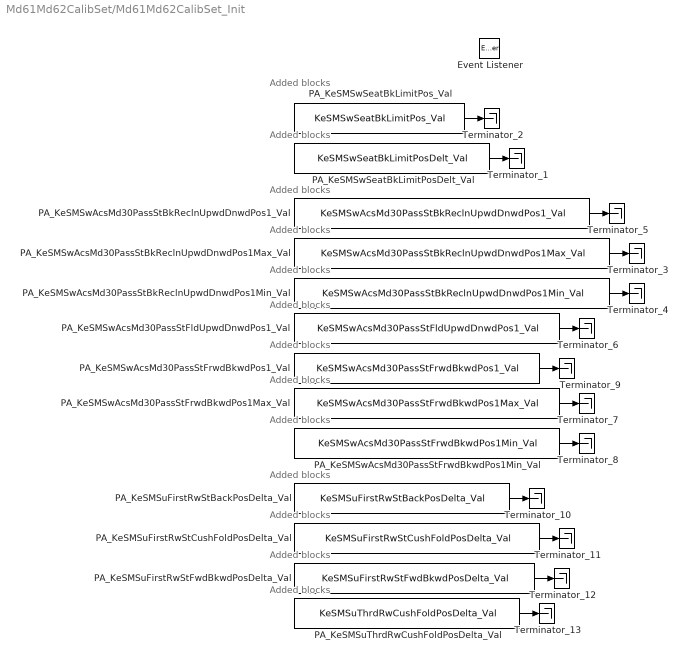
== system Md61Md62CalibSet/Md61Md62CalibSet_Init ==
  note: Added blocks
  note: Added blocks
  note: Added blocks
  note: Added blocks
  note: Added blocks
  note: Added blocks
  note: Added blocks
  note: Added blocks
  note: Added blocks
  note: Added blocks
  note: Added blocks
  note: Added blocks
  note: Added blocks
  Event Listener : EventListener  EventName=reset
  PA_KeSMSuFirstRwStBackPosDelta_Val : Constant  Value=KeSMSuFirstRwStBackPosDelta_Val
  PA_KeSMSuFirstRwStCushFoldPosDelta_Val : Constant  Value=KeSMSuFirstRwStCushFoldPosDelta_Val
  PA_KeSMSuFirstRwStFwdBkwdPosDelta_Val : Constant  Value=KeSMSuFirstRwStFwdBkwdPosDelta_Val
  PA_KeSMSuThrdRwCushFoldPosDelta_Val : Constant  Value=KeSMSuThrdRwCushFoldPosDelta_Val
  PA_KeSMSwAcsMd30PassStBkReclnUpwdDnwdPos1Max_Val : Constant  Value=KeSMSwAcsMd30PassStBkReclnUpwdDnwdPos1Max_Val
  PA_KeSMSwAcsMd30PassStBkReclnUpwdDnwdPos1Min_Val : Constant  Value=KeSMSwAcsMd30PassStBkReclnUpwdDnwdPos1Min_Val
  PA_KeSMSwAcsMd30PassStBkReclnUpwdDnwdPos1_Val : Constant  Value=KeSMSwAcsMd30PassStBkReclnUpwdDnwdPos1_Val
  PA_KeSMSwAcsMd30PassStFldUpwdDnwdPos1_Val : Constant  Value=KeSMSwAcsMd30PassStFldUpwdDnwdPos1_Val
  PA_KeSMSwAcsMd30PassStFrwdBkwdPos1Max_Val : Constant  Value=KeSMSwAcsMd30PassStFrwdBkwdPos1Max_Val
  PA_KeSMSwAcsMd30PassStFrwdBkwdPos1Min_Val : Constant  Value=KeSMSwAcsMd30PassStFrwdBkwdPos1Min_Val
  PA_KeSMSwAcsMd30PassStFrwdBkwdPos1_Val : Constant  Value=KeSMSwAcsMd30PassStFrwdBkwdPos1_Val
  PA_KeSMSwSeatBkLimitPosDelt_Val : Constant  Value=KeSMSwSeatBkLimitPosDelt_Val
  PA_KeSMSwSeatBkLimitPos_Val : Constant  Value=KeSMSwSeatBkLimitPos_Val
  Terminator_{1..13} (13 alike) : Terminator
  wires:
  PA_KeSMSwSeatBkLimitPosDelt_Val/1 -> Terminator_1/1
  PA_KeSMSwSeatBkLimitPos_Val/1 -> Terminator_2/1
  PA_KeSMSwAcsMd30PassStBkReclnUpwdDnwdPos1Max_Val/1 -> Terminator_3/1
  PA_KeSMSwAcsMd30PassStBkReclnUpwdDnwdPos1Min_Val/1 -> Terminator_4/1
  PA_KeSMSwAcsMd30PassStBkReclnUpwdDnwdPos1_Val/1 -> Terminator_5/1
  PA_KeSMSwAcsMd30PassStFldUpwdDnwdPos1_Val/1 -> Terminator_6/1
  PA_KeSMSwAcsMd30PassStFrwdBkwdPos1Max_Val/1 -> Terminator_7/1
  PA_KeSMSwAcsMd30PassStFrwdBkwdPos1Min_Val/1 -> Terminator_8/1
  PA_KeSMSwAcsMd30PassStFrwdBkwdPos1_Val/1 -> Terminator_9/1
  PA_KeSMSuFirstRwStBackPosDelta_Val/1 -> Terminator_10/1
  PA_KeSMSuFirstRwStCushFoldPosDelta_Val/1 -> Terminator_11/1
  PA_KeSMSuFirstRwStFwdBkwdPosDelta_Val/1 -> Terminator_12/1
  PA_KeSMSuThrdRwCushFoldPosDelta_Val/1 -> Terminator_13/1
